simulink model "rtwdemo_reusable"  (Simulink 7.6)
settings: Solver=FixedStepDiscrete  StartTime=0.0  StopTime=10.0  FixedStep=1  RelTol=1e-3
PostLoadFcn:
  | rtwdemo_reusable_data
values from neighbouring files (symbols this model uses):
  k1 = Simulink.Parameter    [rtwdemo_asap2_data.m]
libraries: rtwdemowidgets x2
Description:
  | Reusable Code Interface
settings Model: Creator=The MathWorks Inc.  ExtModeArmWhenConnect=off  ExtModeAutoUpdateStatusClock=off
settings MATStruct: SampleTime=1  Offset=0  Priority=[20.0]
settings DataIOCC: SaveOutput=off  SaveTime=off  SignalLoggingName=sigsOut
settings OptimizationCC: InlineParams=on  InlineInvariantSignals=on  PassReuseOutputArgsAs=Individual arguments  StateBitsets=on  DataBitsets=on  UseTempVars=on  ZeroExternalMemoryAtStartup=off  ZeroInternalMemoryAtStartup=off  NoFixptDivByZeroProtection=on  EfficientFloat2IntCast=on  EfficientMapNaN2IntZero=off  OptimizeModelRefInitCode=on  LifeSpan=1
settings DebuggingCC: CheckExecutionContextPreStartOutputMsg=on  CheckExecutionContextRuntimeOutputMsg=on  SolverPrmCheckMsg=none  UnconnectedInputMsg=none  UnconnectedOutputMsg=none  UnconnectedLineMsg=none  StrictBusMsg=ErrorOnBusTreatedAsVector
settings HardwareCC: ProdIntDivRoundTo=Zero  ProdEndianess=LittleEndian  ProdHWDeviceType=Generic->32-bit Embedded Processor  TargetHWDeviceType=Generic->32-bit Embedded Processor
settings RTWCC: SystemTargetFile=ert.tlc  TLCOptions=-p0 -aWarnNonSaturatedBlocks=0  TemplateMakefile=ert_default_tmf  GenerateReport=on  RTWVerbose=off  ProcessScript=ert_make_rtw_hook  IncludeHyperlinkInReport=on  LaunchReport=on
settings CodeAppCC: ForceParamTrailComments=on  IgnoreCustomStorageClasses=off  IgnoreTestpoints=on  SimulinkDataObjDesc=on  CustomSymbolStrGlobalVar=rt$N$M  CustomSymbolStrType=$N$M  CustomSymbolStrFcn=$N$M$F  CustomSymbolStrMacro=$N$M  InsertBlockDesc=on
settings ERTTargetCC: TargetFcnLib=ansi_tfl_tmw.mat  MultiwordLength=2048  GenerateSampleERTMain=on  IncludeMdlTerminateFcn=off  SupportAbsoluteTime=off  MultiInstanceERTCode=on  SupportNonFinite=off  SupportComplex=off  InlinedParameterPlacement=NonHierarchical  RootIOFormat=Structure reference  ERTCustomFileTemplate=example_file_process.tlc  ConvertIfToSwitch=off

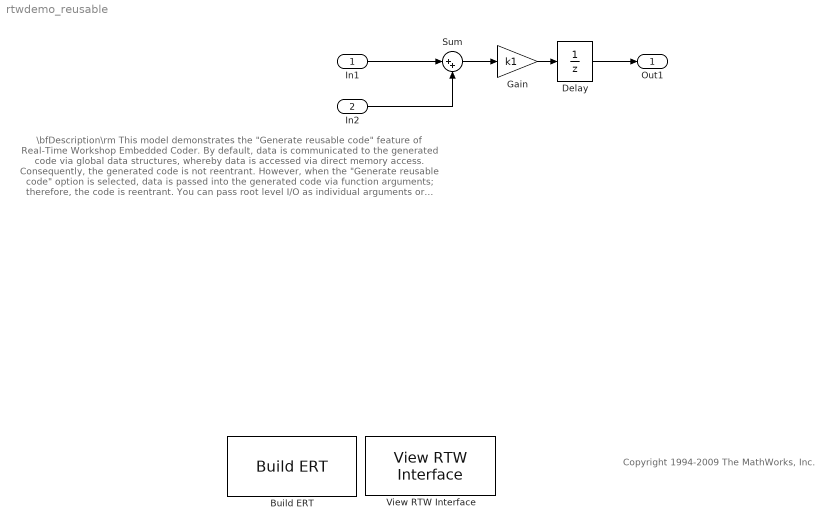
== system rtwdemo_reusable ==
  note: \bfDescription\rm
      | This model demonstrates the "Generate reusable code" feature of Real-Time Workshop
      | Embedded Coder.  By default, data is communicated to the generated code via global data
      | structures, whereby data is accessed via direct memory access.  Consequently, the generated
      | code is not reentrant.  However, when the "Generate reusable code" option is selected,
      | data is passed into the generated code via function arguments; therefore, the code is
      | reentrant.  You can pass root level I/O as individual arguments or packed data structures.
      |
      | \bfInstructions\rm
      | To select the "Generate reusable code" option,
      | 1. From the menu bar, choose Simulation > Configuration Parameters.
      | 2. Select the Real-Time Workshop Interface page.
      | 3. Select the "Generate reusable code" option.
      | 4. Configure the "Reusable code error diagnostic" option.
      | 5. Configure the "Pass root-level I/O as" option.
  note: Copyright 1994-2009 The MathWorks, Inc.
  In1 : Inport  OutDataTypeStr=double  PortDimensions=1  SampleTime=1
  In2 : Inport  Port=2  OutDataTypeStr=double  PortDimensions=1  SampleTime=1
  Build ERT : rtwdemowidgets/Build ERT  SystemSampleTime=-1  attrib_overrides={'MultiInstanceERTCode', 'RootIOFormat'}
  Delay : UnitDelay
  Gain : Gain  Gain=k1  SaturateOnIntegerOverflow=on  OutDataTypeStr=Inherit: Same as input  ParamDataTypeStr=Inherit: Same as input
  Sum : Sum  Inputs=|++  SaturateOnIntegerOverflow=on  InputSameDT=on  OutDataTypeStr=Inherit: Same as first input
  View RTW Interface : rtwdemowidgets/View RTW Interface  SystemSampleTime=-1
  Out1 : Outport
  wires:
  In1/1 -> Sum/1
  Sum/1 -> Gain/1
  In2/1 -> Sum/2
  Gain/1 -> Delay/1
  Delay/1 -> Out1/1
